simulink model "uGrid_1PH_hd_ATD_prueba"  (R2018a)
settings: Solver=ode45  StartTime=0.0  StopTime=1.5  FixedStep=1e-4  MaxStep=1e-4  RelTol=1e-3
PreLoadFcn:
  | SimulinkInit
InitFcn:
  | SimulinkInit
values from neighbouring files (symbols this model uses):
  Ad = sysd.A    [SimulinkInit.m]
  b = 4.91    [parametros_BIO.m]
  Bd = sysd.B    [SimulinkInit.m]
  C = C1+C2+C3+Cl    (= 0.002654)    [SimulinkInit.m]    (also in parametros_BIO.m = 1)
  C1 = Cd(1,:)    [SimulinkInit.m]
  C2 = Cd(2,:)    [SimulinkInit.m]
  C3 = Cd(3,:)    [SimulinkInit.m]
  C4 = Cd(4,:)    [SimulinkInit.m]
  Cd = sysd.C    [SimulinkInit.m]
  K = 25    [parametros_BIO.m]    (also in uio_linear.m = K1+E*H)
  K1 = 1.15    [SimulinkInit.m]    (also in parametros_BIO.m = 9.66; uio_linear.m = K1')
  K11 = 0.8    [parametros_BIO.m]
  K2 = 1    [SimulinkInit.m]    (also in parametros_BIO.m = 6.97)
  K22 = 0.2    [parametros_BIO.m]
  K3 = 1    [SimulinkInit.m]    (also in parametros_BIO.m = 31.8)
  K33 = 0.23    [parametros_BIO.m]
  K4 = 15.1    [parametros_BIO.m]
  Kd = 0.02    [parametros_BIO.m]
  Kdc = 0.02    [parametros_BIO.m]
  Kf = 1    [parametros_BIO.m]
  Kh = 1.2    [parametros_BIO.m]
  Ks = 21.5    [parametros_BIO.m]
  Ksc = 3    [parametros_BIO.m]
  Kv = 1    [parametros_BIO.m]
  Sbin = 13.8    [parametros_BIO.m]
  Svin = 2.91    [parametros_BIO.m]
  T1 = 0.4    [parametros_BIO.m]
  T2 = 1    [parametros_BIO.m]
  T3 = 15    [parametros_BIO.m]
  T4 = 2.5    [parametros_BIO.m]
  T5 = 3.3    [parametros_BIO.m]
  Tao1 = 0.5    [SimulinkInit.m]
  Tcd = 0.2    [parametros_BIO.m]
  Tcr = 0.01    [parametros_BIO.m]
  Tf = 0.04    [parametros_BIO.m]
  tm = 1e-4    (= 0.0001)    [SimulinkInit.m]
  Tr = 950    [parametros_BIO.m]
  Tt = 450    [parametros_BIO.m]
  Ttd = 0.04    [parametros_BIO.m]
  Tv = 0.05    [parametros_BIO.m]
  V = 20    [parametros_BIO.m]
  wref = 70000    [parametros_BIO.m]
  X_acid = 1.2    [parametros_BIO.m]
  X_meth = 0.35    [parametros_BIO.m]
  Z = 3    [parametros_BIO.m]
undefined symbols (not defined in the file or in its folder): F1, F2, F3, F4, G, GF, H1, H2, H3, H4, Ion, K1U, K2U, K3U, K4U, Lithium, ss1, ss2
libraries: powerlib x58, dsparch4 x12, truetime x12, powerlib_meascontrol x4, simulink x1, electricdrivelib x1
(part 3 of 3)

== matlab function uGrid_1PH_hd_ATD_prueba/MeasureNode_I2/MATLAB Function ==
  data: u1 input; y output; u2 input; u3 input
function y = fcn(u1,u2,u3)
t=1;
if (u1>=0.4 && u1<=0.45 || u1>=0.6*1 && u1<=0.66 || u1>=1.19 && u1<=1.26 || u1>=1.35*100 && u1<=1.37) && t==1%u1>=1000
% if (u1>=0.5*1 && u1<=0.6) || (u1>=2*1 && u1<=2.2)|| (u1>=1*100 && u1<=1.3)%u1>=1000
    y=u2+u2*0.25; %0.05
%     y=u3;
else
    y = u2;
    
end

== matlab function uGrid_1PH_hd_ATD_prueba/MeasureNode_I4/MATLAB Function ==
  data: u1 input; y output; u2 input
function y = fcn(u1,u2)
t=1;
if (u1>=0.6 && u1<=0.66 || u1>=0.9 && u1<=0.94 || u1>=1.3 && u1<=1.31) && t==1%u1>=1000
    y=u2+u2*0.3;
else
    y = u2;

end

== matlab function uGrid_1PH_hd_ATD_prueba/MeasureNode_I3/MATLAB Function ==
  data: u1 input; y output; u2 input
function y = fcn(u1,u2)
t=1;
if (u1>=0.10*20 && u1<=0.2*20 || u1>=0.8 && u1<=0.82 || u1>=1.4 && u1<=1.45) && t==1%u1>=1000
    y=u2+u2*0.3;
else
    y = u2;

end

== matlab function uGrid_1PH_hd_ATD_prueba/MeasureNode_I1/MATLAB Function ==
  data: u1 input; y output; u2 input
function y = fcn(u1,u2)
t=1;
if (u1>=0.50 && u1<=0.55 || u1>=0.72 && u1<=0.75 || u1>=1.22 && u1<=1.28) && t==1 %u1>=1000
    y=u2-u2*0.25;
else
    y = u2;

end

== matlab function uGrid_1PH_hd_ATD_prueba/MATLAB Function1 ==
  data: y_hat input; y output; t input
function y = fcn(y_hat,t)%u1,u2,ym1,ym2)
if y_hat(3)>0
    y_hat(3)=y_hat(3)*1.38;
    %     y_hat(3)=y_hat(3)+10;
end

% if t<=0.33
%     y1=y_hat(1)*1;%0.92;
%     y2=y_hat(2)*1;
%     y3=y_hat(3)*1;%1.1; 0.71 0.77 +28
% %     if y3<0
% %         y3=y3+11;
% %     end
%     y4=y_hat(4)*1;%y_hat(4)*1;
%
%
%
% else
%     y1=y_hat(1)*1;%0.92;
%     y2=y_hat(2)*1;
%     y3=y_hat(3)*0.4;%1.1; 0.65; 0.5
%     y4=y_hat(4)*1;%y_hat(4)*1;
% end
if t<=0.33
    y1=y_hat(1)*0.85;
    y2=y_hat(2)*0.8; %0.85
    y3=y_hat(3)*0.57; %0.6
    y4=y_hat(4)*0.88; %0.9
else
    y1=y_hat(1)*0.98;
    y2=y_hat(2)*1.16; %1.13  1.16
    y3=y_hat(3)*0.45; %0.5
    y4=y_hat(4);
    
end

y=[y1 y2 y3 y4];
% if norm_rd >=Th_det
%     rol=1;
% else
%     rol=0;
% end

== matlab function uGrid_1PH_hd_ATD_prueba/MATLAB Function2 ==
  data: r input; y output
function y = fcn(r)%u1,u2,ym1,ym2)

r1=r(1)/2000;%200;
r2=r(2)/2000;%500;
r3=r(3)/2000;%1300;
r4=r(4)/2000;
y=[r1 r2 r3 r4];
% if norm_rd >=Th_det
%     rol=1;
% else
%     rol=0;
% end

== matlab function uGrid_1PH_hd_ATD_prueba/MATLAB Function3 ==
  data: y_hat input; rol output; y_m input; norm_rd output; tiempo input
function [rol,norm_rd] = fcn(y_hat,y_m,tiempo)%u1,u2,ym1,ym2)
Th_det = 6.5e-8;
Th_det=0.07;%2.3e-2; %Funciona bien si los pulsos no estan tan separados
Th_det_up=1;  %2.5 2.25
Th_det_down=-1;
if tiempo >=0.0015 && tiempo <=0.35
    Th_det_up=2.23e-2;  %2.5 2.25
    Th_det_down=3e-4;
else
    Th_det_up=2.25e-2;  %2.5 2.25
    Th_det_down=3e-3;
end
% Th_det=38;
% yol=[u1 ; u2];
% ym=[ym1 ; ym2];

rd1=(y_hat(1)-y_m(1))/100;%200;
rd2=(y_hat(2)-y_m(2))/120;%500;
rd3=(y_hat(3)-y_m(3))/400;%1300; 
rd4=(y_hat(4)-y_m(4))/500;

% rd=y_hat-y_m;
rd=[rd1 rd2 rd3 rd4];
norm_rd=sqrt(sum(rd.^2));
% sys=tf(1,[0.001 1]);


if norm_rd >=Th_det%Th_det_up && norm_rd <=Th_det_down
    rol=1;
else
    rol=0;
end

== matlab function uGrid_1PH_hd_ATD_prueba/MATLAB Function ==
  data: u input; y output; t input
function y = fcn(u,t)
y1=u(1);
y2=u(2);
if t<=0.33
    y3=u(3)*0.69;%*0.52;
else
    y3=u(3)*0.52;
end
y4=u(4);
y5=u(5);
y = [y1 y2 y3 y4 y5];

== matlab function uGrid_1PH_hd_ATD_prueba/MATLAB Function4 ==
  data: u input; y output; t input
function y = fcn(u,t)
y=[0 0 0 0];
if t<=0.04
    y =[0 0 0 0];
else
    y1=u(1)*(10^5)/(10^16);
    y2=u(2)*(10^5)/(10^16);
    y3=u(3)*(10^5)/(10^16);
    y4=u(4)*(10^5)/(10^16);
    y=[y1 y2 y3 y4];
end

== matlab function uGrid_1PH_hd_ATD_prueba/MATLAB Function7 ==
  data: r input; rol output; r1 input; Th_det output
function [rol,Th_det] = fcn(r,r1)%u1,u2,ym1,ym2)
% Th_det = 6.5e-8;
Th_det=0.08;  %2.5

m=r-r1;
if m>0
    Th_det=0.07;%0.1;  %2.5
elseif m<0 && r<=0.007
    Th_det=0.9; 
end


% sys=tf(1,[0.001 1]);


if r >=Th_det
    rol=1;
else
    rol=0;
end

== matlab function uGrid_1PH_hd_ATD_prueba/MATLAB Function14 ==
  data: dr input; r output; t input; ban input; c output; o output
function [r,c,o]   = fcn(dr,t,ban)

if t<=0.33
    th=2e4;
    %     v=2;
else
    th=1e4;
    %     v=3;
end

% r=0;
% c=1;

if ban==1
    r=1;
    c=0;
    if abs(dr(3))>th
        c=1;
        r=0;
    end
else
    r=0;
    c=1;
    if abs(dr(3))>th %%&& ban==0
        c=0;
        r=1;
    end
end

% ra=r;
% a=0;
o=abs(dr(4));

== matlab function uGrid_1PH_hd_ATD_prueba/generador biomasa/MATLAB Function ==
  data: u1 input; y output; u2 input
function y = fcn(u1,u2)

y = u2*(1-u1);

== matlab function uGrid_1PH_hd_ATD_prueba/generador biomasa/MATLAB Function Acetogenesis ==
  data: Xacid input; b input; V input; Ffeed input; um input; Kd input; Ks input; Xacidp output; Sb input
function Xacidp = fcn(Xacid,b,V,Ffeed,um,Kd,Ks,Sb)

% Xacidp=(um/(1+Ks/Sb)-Kd-Ffeed/(b*V))*Xacid;
Xacidp=(um/(Ks/(1+Sb))-Kd-Ffeed/(b*V))*Xacid;

== matlab function uGrid_1PH_hd_ATD_prueba/MATLAB Function6 ==
  data: u input; y output; t input
function y = fcn(u,t)
y=[0 0 0 0];
if t<=0.1
    y =[0 0 0 0];
else
    y1=u(1)*(10^5)/(10^16);
    y2=u(2)*(10^5)/(10^16);
    y3=u(3)*(10^5)/(10^16);
    y4=u(4)*(10^5)/(10^16);
    y=[y1 y2 y3 y4];
end

== matlab function uGrid_1PH_hd_ATD_prueba/generador biomasa/MATLAB Function Acidogenesis ==
  data: Svin input; Sv input; V input; Ffeed input; um input; umc input; K2 input; K3 input; Xacid input; Xmeth input; Ks input; Svp output; Sb input; Ksc input
function Svp = fcn(Svin,Sv,V,Ffeed,um,umc,K2,K3,Xacid,Xmeth,Ks,Sb,Ksc)

% Svp=(Svin-Sv)*(Ffeed/V)+um*K2*Xacid/(1+Ks/Sb)-umc*K3*Xmeth/(1+Ksc/Sv);
Svp=(Svin-Sv)*(Ffeed/V)+um*K2*Xacid/(Ks/(1+Sb))-umc*K3*Xmeth/(Ksc/(1+Sv));

== matlab function uGrid_1PH_hd_ATD_prueba/generador biomasa/MATLAB Function Hidrolisis ==
  data: Sbin input; Sbp output; Sb input; V input; Ffeed input; um input; K1 input; Xacid input; Ks input
function Sbp = fcn(Sbin,Sb,V,Ffeed,um,K1,Xacid,Ks)

% Sbp=(Sbin-Sb)*(Ffeed/V)+um*K1*Xacid/(1+Ks/Sb);
Sbp=(Sbin-Sb)*(Ffeed/V)+um*K1*Xacid/(Ks/(1+Sb));

== matlab function uGrid_1PH_hd_ATD_prueba/generador biomasa/MATLAB Function metano ==
  data: Xmeth input; K4 input; V input; umc input; Ksc input; Sv input; Fmeth output
function Fmeth = fcn(Xmeth,K4,V,umc,Ksc,Sv)


% Fmeth=V*umc*K4*Xmeth/(Ksc/Sv+1);
Fmeth=V*umc*K4*Xmeth/(Ksc/(Sv+1));

== matlab function uGrid_1PH_hd_ATD_prueba/generador biomasa/MATLAB Function metanogenesis ==
  data: Xmeth input; b input; V input; Ffeed input; umc input; Ksc input; Sv input; Xmethp output; Kdc input
function Xmethp = fcn(Xmeth,b,V,Ffeed,umc,Ksc,Sv,Kdc)

% Xmethp=(umc/(Ksc/Sv+1)-Kdc-Ffeed/(b*V))*Xmeth;
Xmethp=(umc/(Ksc/(Sv+1))-Kdc-Ffeed/(b*V))*Xmeth;

== matlab function uGrid_1PH_hd_ATD_prueba/MATLAB Function24 ==
  data: u input; y output; t input
function y = fcn(u,t)
y1=u(1);
y2=u(2);
if t>0.33
    y2=u(2)*1.31;%*0.52;
    y5=u(5)*1.55;
else
    y2=u(2);
    
    y5=u(5)*1.39;
    
end
y3=u(3);
y4=u(4);


y = [y1 y2 y3 y4 y5];

== matlab function uGrid_1PH_hd_ATD_prueba/MATLAB Function25 ==
  data: u input; y output; t input
function y = fcn(u,t)
y1=u(1);
y2=u(2);
if t>0.33
    y3=u(3)*0.54+5;
    y5=u(5)*1.15;
else
    y3=u(3)*0.7;
    
    y5=u(5);
    
end

y4=u(4);


y = [y1 y2 y3 y4 y5];

== matlab function uGrid_1PH_hd_ATD_prueba/MATLAB Function5 ==
  data: u input; y output; t input
function y = fcn(u,t)
y=[0 0 0 0];
if t<=0.3
    y =[0 0 0 0];
else
    y1=u(1)*(10^5)/(10^16);
    y2=u(2)*(10^5)/(10^16);
    y3=u(3)*(10^5)/(10^16);
    y4=u(4)*(10^5)/(10^16);
    y=[y1 y2 y3 y4];
end

== matlab function uGrid_1PH_hd_ATD_prueba/MATLAB Function34 ==
  data: x_hat1 input; v1 output; x_hat2 input; x_hat3 input; x_hat4 input; ruo1 input; rol input
function v1 = fcn(x_hat1,x_hat2,x_hat3,x_hat4,ruo1,rol)

% yol=[u1 ; u2];
% ym=[ym1 ; ym2];
 C1=[0     1     0  0   0];
 v11=C1*(x_hat2'-x_hat1')*ruo1*rol;
 v12=C1*(x_hat2'-x_hat3')*ruo1*rol;
 v13=C1*(x_hat2'-x_hat4')*ruo1*rol;
 
 v1=(v11+v12+v13)/3;

== matlab function uGrid_1PH_hd_ATD_prueba/MATLAB Function38 ==
  data: x_hat1 input; v1 output; x_hat2 input; x_hat3 input; x_hat4 input; ruo1 input; rol input
function v1 = fcn(x_hat1,x_hat2,x_hat3,x_hat4,ruo1,rol)

% yol=[u1 ; u2];
% ym=[ym1 ; ym2];
 C1=[1     0     0  0   0];
 v11=C1*(x_hat1'-x_hat2')*ruo1*rol;
 v12=C1*(x_hat1'-x_hat3')*ruo1*rol;
 v13=C1*(x_hat1'-x_hat4')*ruo1*rol;
 
 v1=(v11+v12+v13)/3;

== matlab function uGrid_1PH_hd_ATD_prueba/MATLAB Function10 ==
  data: u input; y output; t input
function y = fcn(u,t)
y=[0 0 0 0];
if t<=0.3
    y =[0 0 0 0];
else
    y1=u(1)*(10^5)/(10^16);
    y2=u(2)*(10^5)/(10^16);
    y3=u(3)*(10^5)/(10^16);
    y4=u(4)*(10^5)/(10^16);
    y=[y1 y2 y3 y4];
end

== matlab function uGrid_1PH_hd_ATD_prueba/MATLAB Function36 ==
  data: dr input; r output; t input; ban input; c output; o output
function [r,c,o]   = fcn(dr,t,ban)

if t<=0.33
    th=1.5e4;
    %     v=2;
elseif t<=0.55
    th=2e4;
    %     v=3;
else
    th=3e3;
end

% r=0;
% c=1;

if ban==1
    r=1;
    c=0;
    if abs(dr(1))>th
        c=1;
        r=0;
    end
else
    r=0;
    c=1;
    if abs(dr(1))>th %%&& ban==0
        c=0;
        r=1;
    end
end

% ra=r;
% a=0;
o=abs(dr(1));

== matlab function uGrid_1PH_hd_ATD_prueba/MATLAB Function39 ==
  data: x_hat1 input; v1 output; x_hat2 input; x_hat3 input; x_hat4 input; ruo1 input; rol input
function v1 = fcn(x_hat1,x_hat2,x_hat3,x_hat4,ruo1,rol)

% yol=[u1 ; u2];
% ym=[ym1 ; ym2];
 C1=[0     0     1  0   0];
 v11=C1*(x_hat3'-x_hat1')*ruo1*rol;
 v12=C1*(x_hat3'-x_hat2')*ruo1*rol;
 v13=C1*(x_hat3'-x_hat4')*ruo1*rol;
 
 v1=(v11+v12+v13)/3;

== matlab function uGrid_1PH_hd_ATD_prueba/MATLAB Function11 ==
  data: dr input; r output; t input; ban input; c output; o output
function [r,c,o]   = fcn(dr,t,ban)

if t<=0.33
    th=1e4;
    %     v=2;
elseif t<=0.5
    th=1e4;
    %     v=3;
elseif t>0.5 && t<=1
    th=3500;
else
    th=3000;
end

% r=0;
% c=1;

if ban==1
    r=1;
    c=0;
    if abs(dr(2))>th
        c=1;
        r=0;
    end
else
    r=0;
    c=1;
    if abs(dr(2))>th %%&& ban==0
        c=0;
        r=1;
    end
end

% ra=r;
% a=0;
o=abs(dr(2));

== matlab function uGrid_1PH_hd_ATD_prueba/MATLAB Function23 ==
  data: dr input; r output; t input; ban input; c output; o output
function [r,c,o]   = fcn(dr,t,ban)

if t<=0.52
    th=2e4;
    %     v=2;
else
    th=0.7e4;%1e4;
    %     v=3;
end

% r=0;
% c=1;

if ban==1
    r=1;
    c=0;
    if abs(dr(3))>th
        c=1;
        r=0;
    end
else
    r=0;
    c=1;
    if abs(dr(3))>th %%&& ban==0
        c=0;
        r=1;
    end
end

% ra=r;
% a=0;
o=abs(dr(3));
